simulink model "DeltaTest"  (R2018a)
settings: Solver=ode23s  StartTime=0.0  StopTime=50  RelTol=1e-6
settings Model: Creator=augus  LastModifiedBy=augus

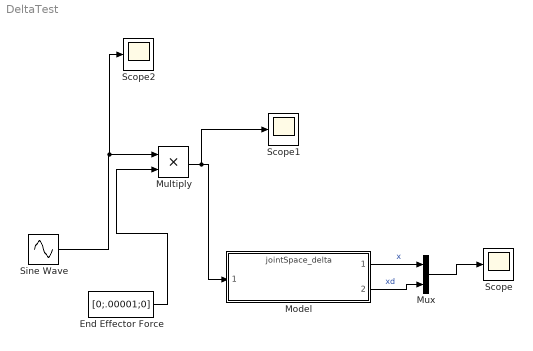
== system DeltaTest ==
  End Effector Force : Constant  Value=[0;.00001;0]
  Model : ModelReference  ModelNameDialog=jointSpace_delta  SimulationMode=Normal  ModelReferenceVersion=1.15
  Multiply : Product
  Mux : Mux  Inputs=2
  Scope : Scope
  Scope1 : Scope
  Scope2 : Scope
  Sine Wave : Sin  SampleTime=0
  wires:
  Multiply/1 -> Scope1/1, Model/1
  Sine Wave/1 -> Scope2/1, Multiply/1
  Model/1 -> Mux/1  "x"
  End Effector Force/1 -> Multiply/2
  Model/2 -> Mux/2  "xd"
  Mux/1 -> Scope/1
